simulink model "NCS_Simulation"  (R2019a)
settings: Solver=ode4  StartTime=0.0  StopTime=200  FixedStep=0.004  MaxStep=0.01  RelTol=1e-3
values from neighbouring files (symbols this model uses):
  CAN2EthernetDelay = 0.000    (= 0)    [Parameter.m]
  CycleTime_Sensor = 1/1000    (= 0.001)    [Parameter.m]
  Ethernet2CANDelay = 0.005    [Parameter.m]
  n = 0.001    [Parameter.m]
  nW_ges = 8    [Parameter.m]
  ReferenceDelay = 0.0    (= 0)    [Parameter.m]
undefined symbols (not defined in the file or in its folder): BUSCapacity, controlGate, entity, m, ReadData, ReadSize, v0
libraries: NCS_Library x250, simulink x12
(part 1 of 3)
settings Model: Creator=Moritz  LastModifiedBy=christophunterauer
settings SolverCC: InitialStep=0.01  MaxConsecutiveZCs=none  ZeroCrossControl=DisableAll  ZeroCrossAlgorithm=Adaptive
settings DataIOCC: ReturnWorkspaceOutputs=off
settings DebuggingCC: ArithmeticOperatorsInVariantConditions=warning

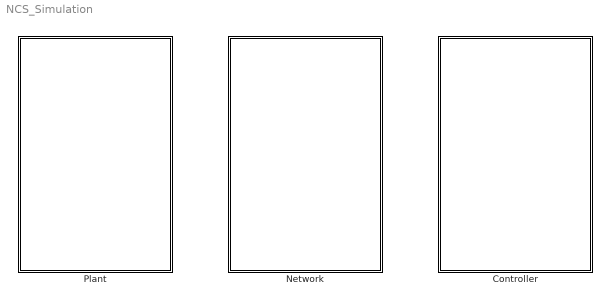
== system NCS_Simulation ==
  Controller : Subsystem
  Network : Subsystem
  Plant : Subsystem

== system NCS_Simulation/Controller ==
  note: k_P = 0.35
  Display : Display
  Display1 : Display
  Subsystem : NCS_Library/Controller/Subsystem  Scenario=Arrival  v_0=300  v_d=300
  Train Controller with PID1 : NCS_Library/Controller/Train Controller with PID  P_dyn=0.5  I_dyn=0  D_dyn=0  P_mg=1  I_mg=0  D_mg=0
  Train Controller with PID2 : NCS_Library/Controller/Train Controller with PID  P_dyn=0.5  I_dyn=0  D_dyn=0  P_mg=1  I_mg=0  D_mg=0
  tag scope: U_1=global, U_2=global
  wires:
  Subsystem/1 -> Train Controller with PID1/2, Train Controller with PID2/2  "Signal"
  Train Controller with PID1/1 -> Display1/1, [U_1]
  [Y_M_1] -> Train Controller with PID1/1  "Y_M"
  [Y_M_2] -> Train Controller with PID2/1  "Y_M"
  Train Controller with PID2/1 -> Display/1, [U_2]

== system NCS_Simulation/Network ==
  Ethernet (Line) : Subsystem  Commented=on
  Ethernet (Line) CAN : Subsystem  Commented=on
  Ethernet (Ring) CAN : Subsystem  Commented=on
  NetworkSelector : NCS_Library/Network/Applications/NetworkSelector  NetworkType=Reference  band=100 MB/s  BER=0.01  RD=0
  Reference : Subsystem

== system NCS_Simulation/Plant ==
  Network to Actuator : Subsystem
  Plant (Train) : Subsystem
  Sensor to Network : Subsystem
  wires:
  Plant (Train)/1(Sensor1) -> Sensor to Network/1(Sensor1)
  Plant (Train)/2(Sensor2) -> Sensor to Network/2(Sensor2)
  Plant (Train)/3(Sensor3) -> Sensor to Network/3(Sensor3)
  Plant (Train)/4(Sensor4) -> Sensor to Network/4(Sensor4)
  Network to Actuator/1(Actuator1) -> Plant (Train)/1(Actuator1)
  Network to Actuator/2(Actuator2) -> Plant (Train)/2(Actuator2)
  Network to Actuator/3(Actuator3) -> Plant (Train)/3(Actuator3)
  Network to Actuator/4(Actuator4) -> Plant (Train)/4(Actuator4)
  Network to Actuator/5(Actuator5) -> Plant (Train)/5(Actuator5)
  Network to Actuator/6(Actuator6) -> Plant (Train)/6(Actuator6)
  Network to Actuator/7(Actuator7) -> Plant (Train)/7(Actuator7)
  Network to Actuator/8(Actuator8) -> Plant (Train)/8(Actuator8)
  Plant (Train)/5(Sensor5) -> Sensor to Network/5(Sensor5)
  Plant (Train)/6(Sensor6) -> Sensor to Network/6(Sensor6)
  Plant (Train)/7(Sensor7) -> Sensor to Network/7(Sensor7)
  Plant (Train)/8(Sensor8) -> Sensor to Network/8(Sensor8)

== system NCS_Simulation/Network/Ethernet (Line) ==
  Consist 1 : Subsystem
  Consist 2 : Subsystem
  Mux Consist : NCS_Library/Network/Applications/Multiplexer/Mux Consist  SystemSampleTime=-1
  tag scope: Ethernet=global
  wires:
  Consist 2/1(out2) -> Mux Consist/2
  Mux Consist/1 -> [Ethernet]
  Consist 1/1(out1) -> Mux Consist/1

== system NCS_Simulation/Network/Ethernet (Line) CAN ==
  Consist 1 : Subsystem
  Consist 2 : Subsystem
  Mux Consist : NCS_Library/Network/Applications/Multiplexer/Mux Consist  SystemSampleTime=-1
  tag scope: CAN=global
  wires:
  Consist 1/1(out1) -> Mux Consist/1
  Mux Consist/1 -> [CAN]
  Consist 2/1(out2) -> Mux Consist/2

== system NCS_Simulation/Network/Ethernet (Ring) CAN ==
  Consist 1 : Subsystem
  Consist 2 : Subsystem
  Mux Consist : NCS_Library/Network/Applications/Multiplexer/Mux Consist  SystemSampleTime=-1
  tag scope: EthernetCAN_Ring=global
  wires:
  Consist 1/1(out1) -> Mux Consist/1
  Mux Consist/1 -> [EthernetCAN_Ring]
  Consist 2/1(out2) -> Mux Consist/2

== system NCS_Simulation/Network/Reference ==
  note: Consist 2
  note: Consist 1
  Mux : NCS_Library/Network/Applications/Multiplexer/Mux  SystemSampleTime=-1
  Mux Consist : NCS_Library/Network/Applications/Multiplexer/Mux Consist  SystemSampleTime=-1
  Mux Reference Y_M : NCS_Library/Network/Applications/Multiplexer/Mux Reference Y_M  SystemSampleTime=-1
  Mux Reference Y_M1 : NCS_Library/Network/Applications/Multiplexer/Mux Reference Y_M  SystemSampleTime=-1
  Mux U : NCS_Library/Network/Applications/Multiplexer/Mux U  SystemSampleTime=-1
  Mux U1 : NCS_Library/Network/Applications/Multiplexer/Mux U  SystemSampleTime=-1
  Mux2 : NCS_Library/Network/Applications/Multiplexer/Mux  SystemSampleTime=-1
  Transport Delay : TransportDelay  DelayTime=ReferenceDelay
  tag scope: Reference=global
  wires:
  Transport Delay/1 -> [Reference]
  [y_M_1] -> Mux Reference Y_M/1
  [y_M_2] -> Mux Reference Y_M/2
  [y_M_3] -> Mux Reference Y_M/3
  [y_M_4] -> Mux Reference Y_M/4
  [y_M_6] -> Mux Reference Y_M1/2
  [y_M_7] -> Mux Reference Y_M1/3
  [y_M_5] -> Mux Reference Y_M1/1
  [y_M_8] -> Mux Reference Y_M1/4
  [U_1] -> Mux U/1
  Mux Reference Y_M/1 -> Mux/1  "Y_M"
  Mux Reference Y_M1/1 -> Mux2/1
  [U_2] -> Mux U1/1
  Mux Consist/1 -> Transport Delay/1
  Mux/1 -> Mux Consist/1
  Mux2/1 -> Mux Consist/2
  Mux U/1 -> Mux/2
  Mux U1/1 -> Mux2/2

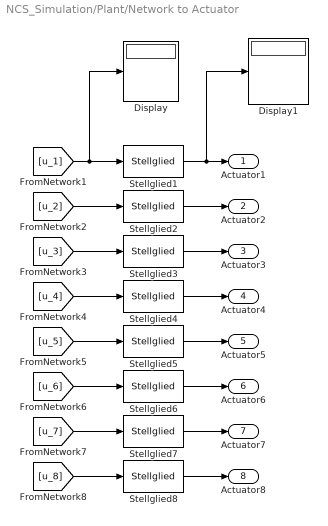
== system NCS_Simulation/Plant/Network to Actuator ==
  Display : Display
  Display1 : Display
  Stellglied{1..8} (8 alike) : NCS_Library/Plant (Train)/Stellglied  SystemSampleTime=-1
  Actuator1 : Outport
  Actuator2 : Outport  Port=2
  Actuator3 : Outport  Port=3
  Actuator4 : Outport  Port=4
  Actuator5 : Outport  Port=5
  Actuator6 : Outport  Port=6
  Actuator7 : Outport  Port=7
  Actuator8 : Outport  Port=8
  wires:
  [u_1] -> Display/1, Stellglied1/1
  [u_4] -> Stellglied4/1
  [u_2] -> Stellglied2/1
  [u_3] -> Stellglied3/1
  Stellglied4/1 -> Actuator4/1
  Stellglied1/1 -> Display1/1, Actuator1/1
  Stellglied2/1 -> Actuator2/1
  Stellglied3/1 -> Actuator3/1
  Stellglied7/1 -> Actuator7/1
  Stellglied6/1 -> Actuator6/1
  Stellglied8/1 -> Actuator8/1
  Stellglied5/1 -> Actuator5/1
  [u_7] -> Stellglied7/1
  [u_5] -> Stellglied5/1
  [u_6] -> Stellglied6/1
  [u_8] -> Stellglied8/1

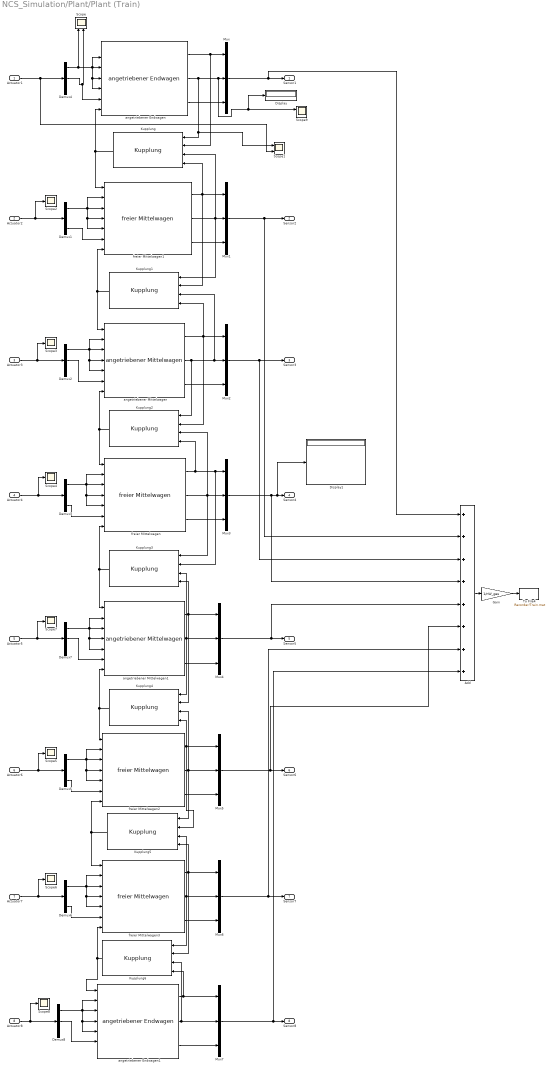
== system NCS_Simulation/Plant/Plant (Train) ==
  Actuator1 : Inport
  Actuator2 : Inport  Port=2
  Actuator3 : Inport  Port=3
  Actuator4 : Inport  Port=4
  Actuator5 : Inport  Port=5
  Actuator6 : Inport  Port=6
  Actuator7 : Inport  Port=7
  Actuator8 : Inport  Port=8
  Add : Sum  Inputs=++++++++
  Demux{1..8} (8 alike) : Demux  Outputs=3
  Display : Display
  Display1 : Display
  Gain : Gain  Gain=1/nW_ges
  Kupplung{,1..6} (7 alike) : NCS_Library/Plant (Train)/Kupplung  SystemSampleTime=-1
  Mux{,1..7} (8 alike) : Mux  Inputs=3
  Scope : Scope  NumInputPorts=2
  Scope1 : Scope  NumInputPorts=2
  Scope{2..8} (7 alike) : Scope
  Scope9 : Scope  NumInputPorts=2
  To File4 : ToFile  Filename=Recorder/Train.mat  MatrixName=Recorder
      mask Display: disp('Recorder')
  angetriebener Endwagen : NCS_Library/Plant (Train)/angetriebener Endwagen  SystemSampleTime=-1
  angetriebener Endwagen1 : NCS_Library/Plant (Train)/angetriebener Endwagen  SystemSampleTime=-1
  angetriebener Mittelwagen : NCS_Library/Plant (Train)/angetriebener Mittelwagen  SystemSampleTime=-1
  angetriebener Mittelwagen1 : NCS_Library/Plant (Train)/angetriebener Mittelwagen  SystemSampleTime=-1
  freier Mittelwagen{,1..3} (4 alike) : NCS_Library/Plant (Train)/freier Mittelwagen  SystemSampleTime=-1
  Sensor1 : Outport
  Sensor2 : Outport  Port=2
  Sensor3 : Outport  Port=3
  Sensor4 : Outport  Port=4
  Sensor5 : Outport  Port=5
  Sensor6 : Outport  Port=6
  Sensor7 : Outport  Port=7
  Sensor8 : Outport  Port=8
  wires:
  Kupplung/1 -> angetriebener Endwagen/7, freier Mittelwagen1/1
  Kupplung2/1 -> freier Mittelwagen/1, angetriebener Mittelwagen/7
  Kupplung1/1 -> freier Mittelwagen1/7, angetriebener Mittelwagen/1
  Demux1/1 -> freier Mittelwagen1/2, freier Mittelwagen1/5, freier Mittelwagen1/4, freier Mittelwagen1/3
  Demux1/3 -> freier Mittelwagen1/6
  Mux/1 -> Add/1, Sensor1/1
  angetriebener Endwagen/2 -> Scope1/1, Kupplung/1, Display/1, Scope9/1, Mux/2
  angetriebener Endwagen/1 -> Kupplung/2, Mux/1
  angetriebener Endwagen/3 -> Mux/3
  freier Mittelwagen1/1 -> Kupplung1/2, Kupplung/4, Mux1/1
  freier Mittelwagen1/2 -> Kupplung1/1, Kupplung/3, Mux1/2
  freier Mittelwagen1/3 -> Mux1/3
  angetriebener Mittelwagen/1 -> Kupplung2/2, Kupplung1/4, Mux2/1
  angetriebener Mittelwagen/2 -> Kupplung2/1, Kupplung1/3, Mux2/2
  angetriebener Mittelwagen/3 -> Mux2/3
  freier Mittelwagen/1 -> Kupplung2/4, Kupplung3/2, Mux3/1
  freier Mittelwagen/2 -> Kupplung3/1, Kupplung2/3, Mux3/2
  freier Mittelwagen/3 -> Mux3/3
  Mux1/1 -> Add/2, Sensor2/1
  Mux2/1 -> Add/3, Sensor3/1
  Mux3/1 -> Add/4, Display1/1, Sensor4/1
  Actuator2/1 -> Scope2/1, Demux1/1
  Demux2/1 -> angetriebener Mittelwagen/5, angetriebener Mittelwagen/4, angetriebener Mittelwagen/2, angetriebener Mittelwagen/3
  Actuator3/1 -> Scope3/1, Demux2/1
  Demux3/1 -> freier Mittelwagen/3, freier Mittelwagen/2, freier Mittelwagen/5, freier Mittelwagen/4
  Demux3/3 -> freier Mittelwagen/6
  Actuator4/1 -> Scope4/1, Demux3/1
  Actuator1/1 -> Scope1/2, Demux4/1
  Demux4/1 -> Scope/1, angetriebener Endwagen/2, angetriebener Endwagen/3, angetriebener Endwagen/5, angetriebener Endwagen/4
  Demux4/2 -> angetriebener Endwagen/6, Scope/2
  Add/1 -> Gain/1
  Gain/1 -> To File4/1
  angetriebener Mittelwagen1/1 -> Mux4/1, Kupplung3/4, Kupplung4/2
  angetriebener Mittelwagen1/2 -> Mux4/2, Kupplung3/3, Kupplung4/1
  Kupplung3/1 -> angetriebener Mittelwagen1/1, freier Mittelwagen/7
  Kupplung4/1 -> angetriebener Mittelwagen1/7, freier Mittelwagen2/1
  Demux5/3 -> freier Mittelwagen2/6
  Actuator6/1 -> Scope5/1, Demux5/1
  Demux5/1 -> freier Mittelwagen2/3, freier Mittelwagen2/2, freier Mittelwagen2/5, freier Mittelwagen2/4
  Demux6/3 -> freier Mittelwagen3/6
  Actuator7/1 -> Scope6/1, Demux6/1
  Demux6/1 -> freier Mittelwagen3/2, freier Mittelwagen3/3, freier Mittelwagen3/4, freier Mittelwagen3/5
  Kupplung5/1 -> freier Mittelwagen3/1, freier Mittelwagen2/7
  Kupplung6/1 -> freier Mittelwagen3/7, angetriebener Endwagen1/1
  freier Mittelwagen3/1 -> Mux6/1, Kupplung5/4, Kupplung6/2
  freier Mittelwagen3/2 -> Mux6/2, Kupplung5/3, Kupplung6/1
  freier Mittelwagen2/2 -> Mux5/2, Kupplung5/1, Kupplung4/3
  freier Mittelwagen2/1 -> Mux5/1, Kupplung5/2, Kupplung4/4
  Actuator5/1 -> Scope7/1, Demux7/1
  Demux7/1 -> angetriebener Mittelwagen1/2, angetriebener Mittelwagen1/3, angetriebener Mittelwagen1/5, angetriebener Mittelwagen1/4
  Demux8/1 -> angetriebener Endwagen1/2, angetriebener Endwagen1/3, angetriebener Endwagen1/5, angetriebener Endwagen1/4
  Actuator8/1 -> Scope8/1, Demux8/1
  angetriebener Endwagen1/1 -> Mux7/1, Kupplung6/4
  Mux4/1 -> Add/5, Sensor5/1
  angetriebener Mittelwagen1/3 -> Mux4/3
  freier Mittelwagen2/3 -> Mux5/3
  Mux5/1 -> Add/6, Sensor6/1
  freier Mittelwagen3/3 -> Mux6/3
  angetriebener Endwagen1/3 -> Mux7/3
  angetriebener Endwagen1/2 -> Mux7/2, Kupplung6/3
  Mux7/1 -> Add/8, Sensor8/1
  Mux6/1 -> Add/7, Sensor7/1
  Demux2/2 -> angetriebener Mittelwagen/6
  Demux7/2 -> angetriebener Mittelwagen1/6
  Demux8/2 -> angetriebener Endwagen1/6

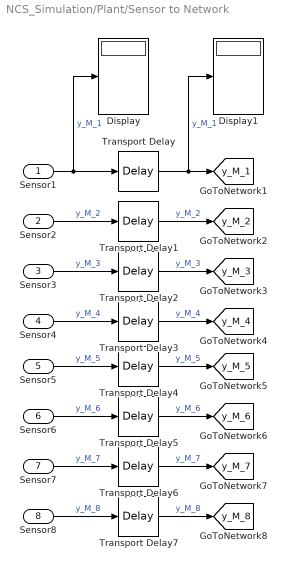
== system NCS_Simulation/Plant/Sensor to Network ==
  Sensor1 : Inport
  Sensor2 : Inport  Port=2
  Sensor3 : Inport  Port=3
  Sensor4 : Inport  Port=4
  Sensor5 : Inport  Port=5
  Sensor6 : Inport  Port=6
  Sensor7 : Inport  Port=7
  Sensor8 : Inport  Port=8
  Display : Display
  Display1 : Display
  Transport Delay{,1..7} (8 alike) : TransportDelay  DelayTime=CycleTime_Sensor  InitialOutput=[ 0 v0 0]
  tag scope: y_M_1=global, y_M_2=global, y_M_3=global, y_M_4=global, y_M_5=global, y_M_6=global, y_M_7=global, y_M_8=global
  wires:
  Sensor1/1 -> Display/1, Transport Delay/1  "y_M_1"
  Transport Delay/1 -> Display1/1, [y_M_1]  "y_M_1"
  Sensor2/1 -> Transport Delay1/1  "y_M_2"
  Sensor3/1 -> Transport Delay2/1  "y_M_3"
  Sensor4/1 -> Transport Delay3/1  "y_M_4"
  Transport Delay1/1 -> [y_M_2]  "y_M_2"
  Transport Delay2/1 -> [y_M_3]  "y_M_3"
  Transport Delay3/1 -> [y_M_4]  "y_M_4"
  Transport Delay7/1 -> [y_M_8]  "y_M_8"
  Transport Delay6/1 -> [y_M_7]  "y_M_7"
  Transport Delay5/1 -> [y_M_6]  "y_M_6"
  Sensor8/1 -> Transport Delay7/1  "y_M_8"
  Sensor7/1 -> Transport Delay6/1  "y_M_7"
  Sensor6/1 -> Transport Delay5/1  "y_M_6"
  Transport Delay4/1 -> [y_M_5]  "y_M_5"
  Sensor5/1 -> Transport Delay4/1  "y_M_5"

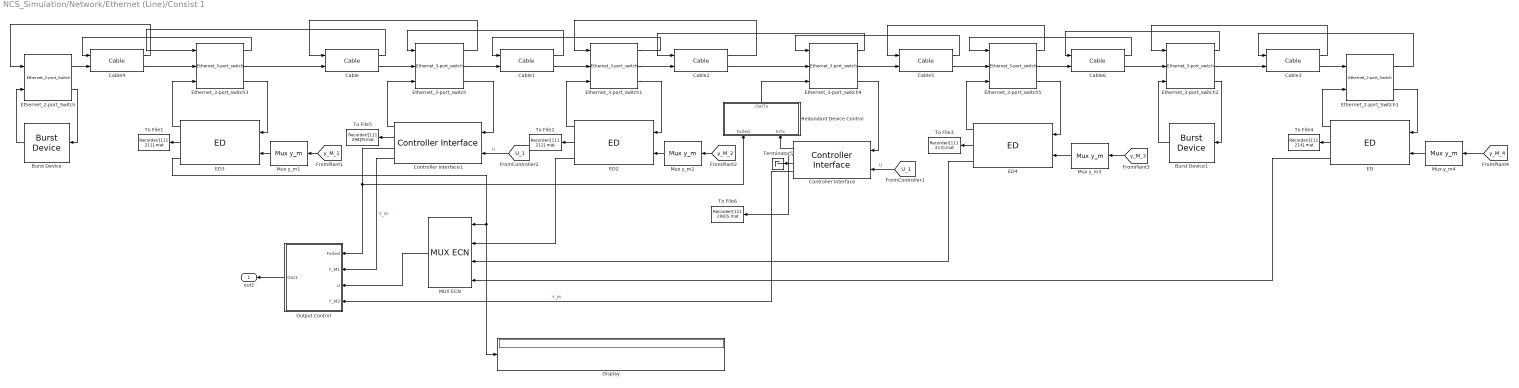
== system NCS_Simulation/Network/Ethernet (Line)/Consist 1 ==
  Burst Device : NCS_Library/Network/ETB/Burst Device  Address=[111 288]  Destination=[ 100 200]  Size=100  Port=1  ReplyAddress=[0 0]  Subscribe=[0 0; 0 0; 0 0; 0 0; 0 0]  msgType=Passive  Tx=0  Timeout=0  SDTv2=Disable  EnableToF=off  ToF=0  EnableBurst=off  ToB=0  n_Burst=0
  Burst Device1 : NCS_Library/Network/ETB/Burst Device  Address=[111 277]  Destination=[ 100 200]  Size=100  Port=1  ReplyAddress=[0 0]  Subscribe=[0 0; 0 0; 0 0; 0 0; 0 0]  msgType=Passive  Tx=0  Timeout=0  SDTv2=Disable  EnableToF=off  ToF=0  EnableBurst=off  ToB=0  n_Burst=0
  Cable{,2,4..6} (5 alike) : NCS_Library/Network/ETB/Cable  length=100  Cable=Coaxial
  Cable1 : NCS_Library/Network/ETB/Cable  length=0  Cable=Coaxial
  Cable3 : NCS_Library/Network/ETB/Cable  length=0  Cable=Coaxial
  Controller Interface : NCS_Library/Network/ETB/Controller Interface  Address=[111 298]  Sensors=[111 211; 111 212; 111 213; 111 214]  Actuators=[111 211; 111 212; 111 213; 111 214]  Size=11  EnableToF=off  ToF=0  Enable_1=on  msgType_1=Push by Controller  SDTv2_1=Disable  Tx_1=40  Enable_2=on  msgType_2=Push by Controller  SDTv2_2=Disable  Tx_2=40  Enable_3=on  msgType_3=Push by Controller  SDTv2_3=Disable  Tx_3=40  Enable_4=on  msgType_4=Push by Controller  SDTv2_4=Disable  Tx_4=40
  Controller Interface1 : NCS_Library/Network/ETB/Controller Interface  Address=[111 298]  Sensors=[111 211; 111 212; 111 213; 111 214]  Actuators=[111 211; 111 212; 111 213; 111 214]  Size=11  EnableToF=off  ToF=0  Enable_1=on  msgType_1=Push by Controller  SDTv2_1=Disable  Tx_1=40  Enable_2=on  msgType_2=Push by Controller  SDTv2_2=Disable  Tx_2=40  Enable_3=on  msgType_3=Push by Controller  SDTv2_3=Disable  Tx_3=40  Enable_4=on  msgType_4=Push by Controller  SDTv2_4=Disable  Tx_4=40
  Display : Display
  ED : NCS_Library/Network/ETB/ED  Address=[111 214]  Destination=[ 111 200 ]  Port=4  ReplyAddress=[0 0]  Size=11  Subscribe=[111 299; 111 298; 0 0; 0 0; 0 0]  msgType=Push cyclical  Tx=40  Timeout=2  SDTv2=Disable  EnableToF=off  ToF=0
  ED2 : NCS_Library/Network/ETB/ED  Address=[111 212]  Destination=[ 111 200]  Port=2  ReplyAddress=[0 0]  Size=11  Subscribe=[111 299; 111 298; 0 0; 0 0; 0 0]  msgType=Push cyclical  Tx=40  Timeout=2  SDTv2=Disable  EnableToF=off  ToF=0
  ED3 : NCS_Library/Network/ETB/ED  Address=[111 211]  Destination=[ 111 200]  Port=1  ReplyAddress=[0 0]  Size=11  Subscribe=[111 299; 111 298; 0 0; 0 0; 0 0]  msgType=Push cyclical  Tx=40  Timeout=2  SDTv2=Disable  EnableToF=off  ToF=5
  ED4 : NCS_Library/Network/ETB/ED  Address=[111 213]  Destination=[ 111 200]  Port=3  ReplyAddress=[0 0]  Size=11  Subscribe=[111 299; 111 298; 0 0; 0 0; 0 0]  msgType=Push cyclical  Tx=40  Timeout=2  SDTv2=Disable  EnableToF=off  ToF=0
  Ethernet_2-port_Switch : NCS_Library/Network/ETB/Ethernet_2-port_Switch  addstore=10  bandc=10^8  buffer_size=120000  cable_node=10  cable_LR=10
  Ethernet_2-port_Switch1 : NCS_Library/Network/ETB/Ethernet_2-port_Switch  addstore=10  bandc=10^8  buffer_size=120000  cable_node=10  cable_LR=10
  Ethernet_3-port_switch{,1..5} (6 alike) : NCS_Library/Network/ETB/Ethernet_3-port_switch  addstore=5  bandc=10^8  buffer_size=180000  cable_node=10  cable_L=10  cable_R=10
  MUX ECN : NCS_Library/Network/Applications/Multiplexer/MUX ECN  SystemSampleTime=-1
  Mux y_m{1..4} (4 alike) : NCS_Library/Network/Applications/Multiplexer/Mux y_m  SystemSampleTime=-1
  Output Control : Subsystem
  Redundant Device Control : Subsystem
  Terminator5 : Terminator
  To File1 : ToFile  Filename=Recorder/[111 211].mat  MatrixName=ED  SaveFormat=Timeseries
  To File2 : ToFile  Filename=Recorder/[111 212].mat  MatrixName=ED  SaveFormat=Timeseries
  To File3 : ToFile  Filename=Recorder/[111 213].mat  MatrixName=ED  SaveFormat=Timeseries
  To File4 : ToFile  Filename=Recorder/[111 214].mat  MatrixName=ED  SaveFormat=Timeseries
  To File5 : ToFile  Filename=Recorder/[111 298]M.mat  MatrixName=ED  SaveFormat=Timeseries
  To File6 : ToFile  Filename=Recorder/[111 298]S.mat  MatrixName=ED  SaveFormat=Timeseries
  out1 : Outport
  wires:
  Controller Interface1/4 -> Output Control/2(Y_M1)  "Y_M"
  Cable3/2 -> Ethernet_2-port_Switch1/1
  Cable2/1 -> Ethernet_3-port_switch1/1
  Controller Interface/1 -> Redundant Device Control/2(InTx)
  Ethernet_2-port_Switch/2 -> Burst Device/1
  Ethernet_2-port_Switch1/1 -> Cable3/1
  Burst Device/1 -> Ethernet_2-port_Switch/2
  Ethernet_3-port_switch/3 -> Controller Interface1/1
  Controller Interface1/3 -> Redundant Device Control/1(Failed), Output Control/1(Failed)
  Cable1/1 -> Ethernet_3-port_switch/1
  Controller Interface/4 -> Output Control/4(Y_M2)  "Y_M"
  Ethernet_3-port_switch/1 -> Cable/1
  Cable3/1 -> Ethernet_3-port_switch2/1
  Output Control/1(Out1) -> out1/1
  [U_1] -> Controller Interface/2  "U"
  Ethernet_3-port_switch2/2 -> Cable3/2
  Ethernet_3-port_switch1/2 -> Cable2/2
  Ethernet_3-port_switch/2 -> Cable1/2
  Cable/2 -> Ethernet_3-port_switch/2
  Cable1/2 -> Ethernet_3-port_switch1/2
  Ethernet_3-port_switch1/1 -> Cable1/1
  Controller Interface1/1 -> Ethernet_3-port_switch/3
  [U_1] -> Controller Interface1/2  "U"
  ED2/1 -> Ethernet_3-port_switch1/3
  Ethernet_3-port_switch1/3 -> ED2/1
  ED2/2 -> To File2/1
  [y_M_2] -> Mux y_m2/1
  Ethernet_3-port_switch3/2 -> Cable/2
  Cable/1 -> Ethernet_3-port_switch3/1
  ED3/1 -> Ethernet_3-port_switch3/3
  Ethernet_3-port_switch3/3 -> ED3/1
  Ethernet_2-port_Switch/1 -> Cable4/2
  Cable4/2 -> Ethernet_3-port_switch3/2
  Cable4/1 -> Ethernet_2-port_Switch/1
  Ethernet_3-port_switch3/1 -> Cable4/1
  Cable2/2 -> Ethernet_3-port_switch4/2
  Ethernet_3-port_switch4/2 -> Cable5/2
  Cable5/2 -> Ethernet_3-port_switch5/2
  Redundant Device Control/1(OutTx) -> Ethernet_3-port_switch4/3
  Ethernet_3-port_switch4/3 -> Controller Interface/1
  ED4/1 -> Ethernet_3-port_switch5/3
  Ethernet_3-port_switch5/3 -> ED4/1
  [y_M_3] -> Mux y_m3/1
  ED4/2 -> To File3/1
  Ethernet_3-port_switch5/2 -> Cable6/2
  Cable6/2 -> Ethernet_3-port_switch2/2
  Ethernet_3-port_switch4/1 -> Cable2/1
  Cable5/1 -> Ethernet_3-port_switch4/1
  Ethernet_3-port_switch5/1 -> Cable5/1
  Ethernet_3-port_switch2/3 -> Burst Device1/1
  Burst Device1/1 -> Ethernet_3-port_switch2/3
  Cable6/1 -> Ethernet_3-port_switch5/1
  Ethernet_3-port_switch2/1 -> Cable6/1
  ED/1 -> Ethernet_2-port_Switch1/2
  Ethernet_2-port_Switch1/2 -> ED/1
  ED/2 -> To File4/1
  [y_M_4] -> Mux y_m4/1
  [y_M_1] -> Mux y_m1/1
  ED3/2 -> To File1/1
  Controller Interface/2 -> To File6/1
  MUX ECN/1 -> Output Control/3(U)
  ED3/3 -> Display/1, MUX ECN/1
  ED2/3 -> MUX ECN/2
  ED4/3 -> MUX ECN/3
  ED/3 -> MUX ECN/4
  Mux y_m1/1 -> ED3/2
  Mux y_m4/1 -> ED/2
  Mux y_m3/1 -> ED4/2
  Mux y_m2/1 -> ED2/2
  Controller Interface/3 -> Terminator5/1
  Controller Interface1/2 -> To File5/1

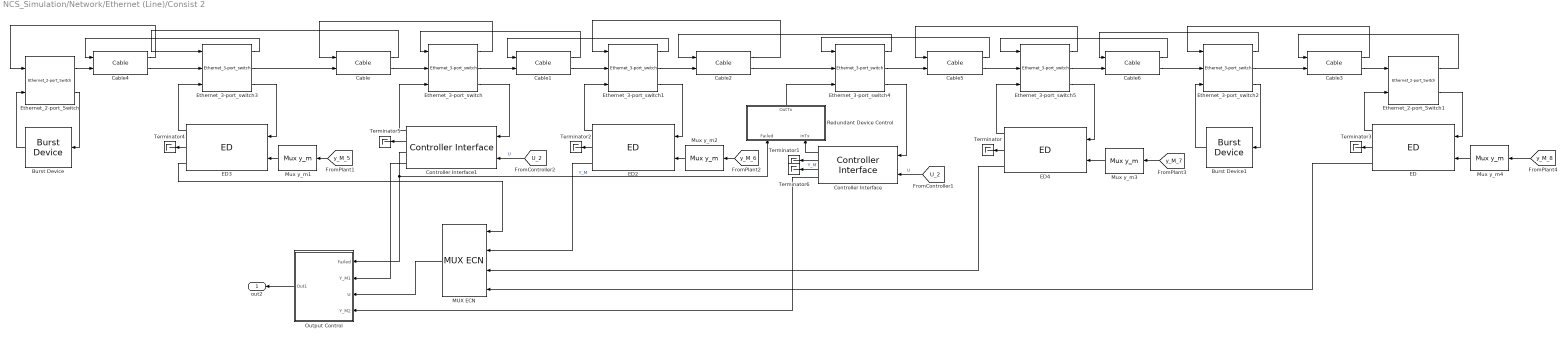
== system NCS_Simulation/Network/Ethernet (Line)/Consist 2 ==
  Burst Device : NCS_Library/Network/ETB/Burst Device  Address=[111 288]  Destination=[ 100 200]  Size=100  Port=1  ReplyAddress=[0 0]  Subscribe=[0 0; 0 0; 0 0; 0 0; 0 0]  msgType=Passive  Tx=0  Timeout=0  SDTv2=Disable  EnableToF=off  ToF=0  EnableBurst=off  ToB=0  n_Burst=0
  Burst Device1 : NCS_Library/Network/ETB/Burst Device  Address=[111 277]  Destination=[ 100 200]  Size=100  Port=1  ReplyAddress=[0 0]  Subscribe=[0 0; 0 0; 0 0; 0 0; 0 0]  msgType=Passive  Tx=0  Timeout=0  SDTv2=Disable  EnableToF=off  ToF=0  EnableBurst=on  ToB=30  n_Burst=10000
  Cable{,2,4..6} (5 alike) : NCS_Library/Network/ETB/Cable  length=100  Cable=Coaxial
  Cable1 : NCS_Library/Network/ETB/Cable  length=0  Cable=Coaxial
  Cable3 : NCS_Library/Network/ETB/Cable  length=0  Cable=Coaxial
  Controller Interface : NCS_Library/Network/ETB/Controller Interface  Address=[111 298]  Sensors=[111 211; 111 212; 111 213; 111 214]  Actuators=[111 211; 111 212; 111 213; 111 214]  Size=11  EnableToF=off  ToF=0  Enable_1=on  msgType_1=Push by Controller  SDTv2_1=Disable  Tx_1=0.1  Enable_2=on  msgType_2=Push by Controller  SDTv2_2=Disable  Tx_2=0.1  Enable_3=on  msgType_3=Push by Controller  SDTv2_3=Disable  Tx_3=0.1  Enable_4=on  msgType_4=Push by Controller  SDTv2_4=Disable  Tx_4=0.1
  Controller Interface1 : NCS_Library/Network/ETB/Controller Interface  Address=[111 299]  Sensors=[111 211; 111 212; 111 213; 111 214]  Actuators=[111 211; 111 212; 111 213; 111 214]  Size=11  EnableToF=off  ToF=0  Enable_1=on  msgType_1=Push by Controller  SDTv2_1=Disable  Tx_1=40  Enable_2=on  msgType_2=Push by Controller  SDTv2_2=Disable  Tx_2=40  Enable_3=on  msgType_3=Push by Controller  SDTv2_3=Disable  Tx_3=40  Enable_4=on  msgType_4=Push by Controller  SDTv2_4=Disable  Tx_4=40
  ED : NCS_Library/Network/ETB/ED  Address=[111 214]  Destination=[ 111 200 ]  Port=4  ReplyAddress=[0 0]  Size=11  Subscribe=[111 299; 111 298; 0 0; 0 0; 0 0]  msgType=Push cyclical  Tx=40  Timeout=2  SDTv2=Disable  EnableToF=off  ToF=0
  ED2 : NCS_Library/Network/ETB/ED  Address=[111 212]  Destination=[ 111 200]  Port=2  ReplyAddress=[0 0]  Size=11  Subscribe=[111 299; 111 298; 0 0; 0 0; 0 0]  msgType=Push cyclical  Tx=40  Timeout=2  SDTv2=Disable  EnableToF=off  ToF=0
  ED3 : NCS_Library/Network/ETB/ED  Address=[111 211]  Destination=[ 111 200]  Port=1  ReplyAddress=[0 0]  Size=11  Subscribe=[111 299; 111 298; 0 0; 0 0; 0 0]  msgType=Push cyclical  Tx=40  Timeout=2  SDTv2=Disable  EnableToF=off  ToF=0
  ED4 : NCS_Library/Network/ETB/ED  Address=[111 213]  Destination=[ 111 200]  Port=3  ReplyAddress=[0 0]  Size=11  Subscribe=[111 299; 111 298; 0 0; 0 0; 0 0]  msgType=Push cyclical  Tx=40  Timeout=2  SDTv2=Disable  EnableToF=off  ToF=0
  Ethernet_2-port_Switch : NCS_Library/Network/ETB/Ethernet_2-port_Switch  addstore=10  bandc=10^8  buffer_size=120000  cable_node=10  cable_LR=10
  Ethernet_2-port_Switch1 : NCS_Library/Network/ETB/Ethernet_2-port_Switch  addstore=10  bandc=10^8  buffer_size=120000  cable_node=10  cable_LR=10
  Ethernet_3-port_switch{,1..5} (6 alike) : NCS_Library/Network/ETB/Ethernet_3-port_switch  addstore=5  bandc=10^8  buffer_size=180000  cable_node=10  cable_L=10  cable_R=10
  MUX ECN : NCS_Library/Network/Applications/Multiplexer/MUX ECN  SystemSampleTime=-1
  Mux y_m{1..4} (4 alike) : NCS_Library/Network/Applications/Multiplexer/Mux y_m  SystemSampleTime=-1
  Output Control : Subsystem
  Redundant Device Control : Subsystem
  Terminator{,1..6} (7 alike) : Terminator
  out2 : Outport
  wires:
  Cable3/2 -> Ethernet_2-port_Switch1/1
  Cable2/1 -> Ethernet_3-port_switch1/1
  Controller Interface/1 -> Redundant Device Control/2(InTx)
  Ethernet_2-port_Switch/2 -> Burst Device/1
  Ethernet_2-port_Switch1/1 -> Cable3/1
  Burst Device/1 -> Ethernet_2-port_Switch/2
  Ethernet_3-port_switch/3 -> Controller Interface1/1
  Cable1/1 -> Ethernet_3-port_switch/1
  Ethernet_3-port_switch/1 -> Cable/1
  Cable3/1 -> Ethernet_3-port_switch2/1
  Output Control/1(Out1) -> out2/1
  [U_2] -> Controller Interface/2  "U"
  Ethernet_3-port_switch2/2 -> Cable3/2
  Ethernet_3-port_switch1/2 -> Cable2/2
  Ethernet_3-port_switch/2 -> Cable1/2
  Cable/2 -> Ethernet_3-port_switch/2
  Cable1/2 -> Ethernet_3-port_switch1/2
  Ethernet_3-port_switch1/1 -> Cable1/1
  Controller Interface1/1 -> Ethernet_3-port_switch/3
  [U_2] -> Controller Interface1/2  "U"
  ED2/1 -> Ethernet_3-port_switch1/3
  Ethernet_3-port_switch1/3 -> ED2/1
  ED2/2 -> Terminator2/1
  [y_M_6] -> Mux y_m2/1
  Ethernet_3-port_switch3/2 -> Cable/2
  Cable/1 -> Ethernet_3-port_switch3/1
  ED3/1 -> Ethernet_3-port_switch3/3
  Ethernet_3-port_switch3/3 -> ED3/1
  Ethernet_2-port_Switch/1 -> Cable4/2
  Cable4/2 -> Ethernet_3-port_switch3/2
  Cable4/1 -> Ethernet_2-port_Switch/1
  Ethernet_3-port_switch3/1 -> Cable4/1
  Cable2/2 -> Ethernet_3-port_switch4/2
  Ethernet_3-port_switch4/2 -> Cable5/2
  Cable5/2 -> Ethernet_3-port_switch5/2
  Redundant Device Control/1(OutTx) -> Ethernet_3-port_switch4/3
  Ethernet_3-port_switch4/3 -> Controller Interface/1
  ED4/1 -> Ethernet_3-port_switch5/3
  Ethernet_3-port_switch5/3 -> ED4/1
  [y_M_7] -> Mux y_m3/1
  ED4/2 -> Terminator/1
  Ethernet_3-port_switch5/2 -> Cable6/2
  Cable6/2 -> Ethernet_3-port_switch2/2
  Ethernet_3-port_switch4/1 -> Cable2/1
  Cable5/1 -> Ethernet_3-port_switch4/1
  Ethernet_3-port_switch5/1 -> Cable5/1
  Ethernet_3-port_switch2/3 -> Burst Device1/1
  Burst Device1/1 -> Ethernet_3-port_switch2/3
  Cable6/1 -> Ethernet_3-port_switch5/1
  Ethernet_3-port_switch2/1 -> Cable6/1
  ED/1 -> Ethernet_2-port_Switch1/2
  Ethernet_2-port_Switch1/2 -> ED/1
  ED/2 -> Terminator3/1
  [y_M_8] -> Mux y_m4/1
  [y_M_5] -> Mux y_m1/1
  ED3/2 -> Terminator4/1
  Controller Interface/2 -> Terminator1/1
  MUX ECN/1 -> Output Control/3(U)
  ED3/3 -> MUX ECN/1
  ED2/3 -> MUX ECN/2
  ED4/3 -> MUX ECN/3
  ED/3 -> MUX ECN/4
  Mux y_m1/1 -> ED3/2
  Mux y_m4/1 -> ED/2
  Mux y_m3/1 -> ED4/2
  Mux y_m2/1 -> ED2/2
  Controller Interface1/4 -> Output Control/2(Y_M1)
  Controller Interface1/3 -> Output Control/1(Failed), Redundant Device Control/1(Failed)  "Y_M"
  Controller Interface1/2 -> Terminator5/1
  Controller Interface/4 -> Output Control/4(Y_M2)
  Controller Interface/3 -> Terminator6/1  "Y_M"

== system NCS_Simulation/Network/Ethernet (Line) CAN/Consist 1 ==
  Burst Device : NCS_Library/Network/ETB/Burst Device  Address=[111 299]  Destination=[ 100 200]  Port=1  ReplyAddress=[0 0]  Subscribe=[0 0; 0 0; 0 0; 0 0; 0 0]  msgType=Passive  Tx=0  Timeout=0  SDTv2=Disable  EnableToF=off  ToF=0  EnableBurst=off  ToB=0  n_Burst=0
  Burst Device1 : NCS_Library/Network/ETB/Burst Device  Address=[111 298]  Destination=[ 100 200]  Port=1  ReplyAddress=[0 0]  Subscribe=[0 0; 0 0; 0 0; 0 0; 0 0]  msgType=Passive  Tx=0  Timeout=0  SDTv2=Disable  EnableToF=off  ToF=0  EnableBurst=off  ToB=0  n_Burst=0
  Bus Selector : BusSelector  OutputSignals=#Receive
  Cable{,1..3} (4 alike) : NCS_Library/Network/ETB/Cable  length=0  Cable=Coaxial
  ED : NCS_Library/Network/ETB/ED  Address=[111 212]  Destination=[111 211]  Port=1  ReplyAddress=[0 0]  Size=11  Subscribe=[111 211; 0 0; 0 0; 0 0; 0 0]  msgType=Passive  Tx=0.1  Timeout=inf  SDTv2=Disable  EnableToF=on  ToF=6
  ED1 : NCS_Library/Network/ETB/ED  Address=[111 213]  Destination=[111 211]  Port=1  ReplyAddress=[0 0]  Size=11  Subscribe=[111 211; 0 0; 0 0; 0 0; 0 0]  msgType=Passive  Tx=0.1  Timeout=inf  SDTv2=Disable  EnableToF=off  ToF=0.5
  Ethernet_2-port_Switch : NCS_Library/Network/ETB/Ethernet_2-port_Switch  addstore=10  bandc=10^8  buffer_size=120000  cable_node=10  cable_LR=10
  Ethernet_2-port_Switch1 : NCS_Library/Network/ETB/Ethernet_2-port_Switch  addstore=10  bandc=10^8  buffer_size=120000  cable_node=10  cable_LR=10
  Ethernet_3-port_switch : NCS_Library/Network/ETB/Ethernet_3-port_switch  addstore=5  bandc=10^8  buffer_size=180000  cable_node=10  cable_L=10  cable_R=10
  Ethernet_3-port_switch1 : NCS_Library/Network/ETB/Ethernet_3-port_switch  addstore=5  bandc=10^8  buffer_size=180000  cable_node=10  cable_L=10  cable_R=10
  Ethernet_3-port_switch2 : NCS_Library/Network/ETB/Ethernet_3-port_switch  addstore=5  bandc=10^8  buffer_size=180000  cable_node=10  cable_L=10  cable_R=10
  Fieldbus 1 : Subsystem
  Output Control : Subsystem
  Redundant Device Control : Subsystem
  Terminator1 : Terminator
  out1 : Outport
  wires:
  [U_1] -> ED/2  "U"
  ED/1 -> Ethernet_3-port_switch/3
  ED/2 -> Bus Selector/1
  ED1/2 -> Terminator1/1
  Ethernet_3-port_switch1/1 -> Cable1/1
  Cable1/2 -> Ethernet_3-port_switch1/2
  Ethernet_2-port_Switch/1 -> Cable/2
  Cable/2 -> Ethernet_3-port_switch/2
  Ethernet_3-port_switch/2 -> Cable1/2
  Ethernet_3-port_switch1/2 -> Cable2/2
  Ethernet_3-port_switch2/2 -> Cable3/2
  [U_1] -> ED1/2  "U"
  Output Control/1(Out1) -> out1/1
  Cable3/1 -> Ethernet_3-port_switch2/1
  Ethernet_3-port_switch/1 -> Cable/1
  Redundant Device Control/1(OutTx) -> Ethernet_3-port_switch2/3
  ED1/3 -> Output Control/4(Y_M2)  "Y_M"
  Ethernet_3-port_switch2/1 -> Cable2/1
  Ethernet_2-port_Switch1/2 -> Burst Device1/1
  Ethernet_3-port_switch1/3 -> Fieldbus 1/1(InFromEthernet)
  Fieldbus 1/1(OutToEthernet) -> Ethernet_3-port_switch1/3
  Ethernet_3-port_switch2/3 -> ED1/1
  Burst Device1/1 -> Ethernet_2-port_Switch1/2
  Cable1/1 -> Ethernet_3-port_switch/1
  Bus Selector/1 -> Output Control/1(<#Receive>), Redundant Device Control/1(<#Receive>)  "<#Receive>"
  Cable/1 -> Ethernet_2-port_Switch/1
  Ethernet_3-port_switch/3 -> ED/1
  Burst Device/1 -> Ethernet_2-port_Switch/2
  Ethernet_2-port_Switch1/1 -> Cable3/1
  Cable2/2 -> Ethernet_3-port_switch2/2
  Ethernet_2-port_Switch/2 -> Burst Device/1
  ED1/1 -> Redundant Device Control/2(InTx)
  Cable2/1 -> Ethernet_3-port_switch1/1
  Cable3/2 -> Ethernet_2-port_Switch1/1
  ED/3 -> Output Control/2(Y_M1)  "Y_M"
  Fieldbus 1/2(U) -> Output Control/3(U)  "U"

== system NCS_Simulation/Network/Ethernet (Line) CAN/Consist 2 ==
  Burst Device : NCS_Library/Network/ETB/Burst Device  Address=[111 299]  Destination=[ 100 200]  Port=1  ReplyAddress=[0 0]  Subscribe=[0 0; 0 0; 0 0; 0 0; 0 0]  msgType=Passive  Tx=0  Timeout=0  SDTv2=Disable  EnableToF=off  ToF=0  EnableBurst=off  ToB=0  n_Burst=0
  Burst Device1 : NCS_Library/Network/ETB/Burst Device  Address=[111 298]  Destination=[ 100 200]  Port=1  ReplyAddress=[0 0]  Subscribe=[0 0; 0 0; 0 0; 0 0; 0 0]  msgType=Passive  Tx=0  Timeout=0  SDTv2=Disable  EnableToF=off  ToF=0  EnableBurst=off  ToB=0  n_Burst=0
  Bus Selector : BusSelector  OutputSignals=#Receive
  Cable{,1..3} (4 alike) : NCS_Library/Network/ETB/Cable  length=0  Cable=Coaxial
  ED : NCS_Library/Network/ETB/ED  Address=[112 212]  Destination=[112 211]  Port=1  ReplyAddress=[0 0]  Subscribe=[112 211; 0 0; 0 0; 0 0; 0 0]  msgType=Push Continuous  Tx=0.1  Timeout=inf  SDTv2=Disable  EnableToF=off  ToF=6  EnableBurst=off  ToB=0
  ED1 : NCS_Library/Network/ETB/ED  Address=[112 213]  Destination=[112 211]  Port=1  ReplyAddress=[0 0]  Subscribe=[112 211; 0 0; 0 0; 0 0; 0 0]  msgType=Push Continuous  Tx=0.1  Timeout=inf  SDTv2=Disable  EnableToF=off  ToF=0.5  EnableBurst=off  ToB=0
  Ethernet_2-port_Switch : NCS_Library/Network/ETB/Ethernet_2-port_Switch  addstore=10  bandc=10^8  buffer_size=120000  cable_node=10  cable_LR=10
  Ethernet_2-port_Switch1 : NCS_Library/Network/ETB/Ethernet_2-port_Switch  addstore=10  bandc=10^8  buffer_size=120000  cable_node=10  cable_LR=10
  Ethernet_3-port_switch : NCS_Library/Network/ETB/Ethernet_3-port_switch  addstore=5  bandc=10^8  buffer_size=180000  cable_node=10  cable_L=10  cable_R=10
  Ethernet_3-port_switch1 : NCS_Library/Network/ETB/Ethernet_3-port_switch  addstore=5  bandc=10^8  buffer_size=180000  cable_node=10  cable_L=10  cable_R=10
  Ethernet_3-port_switch2 : NCS_Library/Network/ETB/Ethernet_3-port_switch  addstore=5  bandc=10^8  buffer_size=180000  cable_node=10  cable_L=10  cable_R=10
  Fieldbus 2 : Subsystem
  Output Control : Subsystem
  Redundant Device Control : Subsystem
  Terminator1 : Terminator
  out2 : Outport
  wires:
  Fieldbus 2/2(U) -> Output Control/3(U)  "U"
  ED/3 -> Output Control/2(Y_M1)  "Y_M"
  Cable3/2 -> Ethernet_2-port_Switch1/1
  Cable2/1 -> Ethernet_3-port_switch1/1
  ED1/1 -> Redundant Device Control/2(InTx)
  Ethernet_2-port_Switch/2 -> Burst Device/1
  Cable2/2 -> Ethernet_3-port_switch2/2
  Ethernet_2-port_Switch1/1 -> Cable3/1
  Burst Device/1 -> Ethernet_2-port_Switch/2
  Ethernet_3-port_switch/3 -> ED/1
  Cable/1 -> Ethernet_2-port_Switch/1
  Bus Selector/1 -> Redundant Device Control/1(<#Receive>), Output Control/1(<#Receive>)  "<#Receive>"
  Cable1/1 -> Ethernet_3-port_switch/1
  Burst Device1/1 -> Ethernet_2-port_Switch1/2
  Ethernet_3-port_switch2/3 -> ED1/1
  Fieldbus 2/1(OutToEthernet) -> Ethernet_3-port_switch1/3
  Ethernet_3-port_switch1/3 -> Fieldbus 2/1(InFromEthernet)
  Ethernet_2-port_Switch1/2 -> Burst Device1/1
  Ethernet_3-port_switch2/1 -> Cable2/1
  ED1/3 -> Output Control/4(Y_M2)  "Y_M"
  Redundant Device Control/1(OutTx) -> Ethernet_3-port_switch2/3
  Ethernet_3-port_switch/1 -> Cable/1
  Cable3/1 -> Ethernet_3-port_switch2/1
  Output Control/1(Out1) -> out2/1
  Ethernet_3-port_switch2/2 -> Cable3/2
  Ethernet_3-port_switch1/2 -> Cable2/2
  Ethernet_3-port_switch/2 -> Cable1/2
  Cable/2 -> Ethernet_3-port_switch/2
  Ethernet_2-port_Switch/1 -> Cable/2
  Cable1/2 -> Ethernet_3-port_switch1/2
  Ethernet_3-port_switch1/1 -> Cable1/1
  ED1/2 -> Terminator1/1
  ED/2 -> Bus Selector/1
  ED/1 -> Ethernet_3-port_switch/3
  [U_2] -> ED/2  "U"
  [U_2] -> ED1/2  "U"

== system NCS_Simulation/Network/Ethernet (Ring) CAN/Consist 1 ==
  Burst Device : NCS_Library/Network/ETB/Burst Device  Address=[111 299]  Destination=[ 100 200]  Size=100  Port=1  ReplyAddress=[0 0]  Subscribe=[0 0; 0 0; 0 0; 0 0; 0 0]  msgType=Passive  T_x=0  Timeout=0  SDTv2=Disable  EnableToF=off  ToF=0  EnableBurst=off  ToB=0  Tx=0  number=1
  Burst Device1 : NCS_Library/Network/ETB/Burst Device  Address=[111 298]  Destination=[ 100 200]  Size=100  Port=1  ReplyAddress=[0 0]  Subscribe=[0 0; 0 0; 0 0; 0 0; 0 0]  msgType=Passive  T_x=0  Timeout=0  SDTv2=Disable  EnableToF=off  ToF=0  EnableBurst=off  ToB=0  Tx=0  number=1
  Cable{,1..4} (5 alike) : NCS_Library/Network/ETB/Cable  length=0  Cable=Coaxial
  Controller Interface : NCS_Library/Network/ETB/Controller Interface  Address=[144 211]  Sensors=[133 211; 0 0; 0 0; 0 0]  Actuators=[133 211; 0 0; 0 0; 0 0]  Size=11  EnableToF=off  ToF=0  Enable_1=on  msgType_1=Push by Controller  SDTv2_1=Disable  Tx_1=0.1  Enable_2=off  msgType_2=Push by Controller  SDTv2_2=Disable  Tx_2=0  Enable_3=off  msgType_3=Push by Controller  SDTv2_3=Disable  Tx_3=0  Enable_4=off  msgType_4=Push by Controller  SDTv2_4=Disable  Tx_4=0
  Controller Interface1 : NCS_Library/Network/ETB/Controller Interface  Address=[122 211]  Sensors=[133 211; 0 0; 0 0; 0 0]  Actuators=[133 211; 0 0; 0 0; 0 0]  Size=11  EnableToF=off  ToF=0  Enable_1=on  msgType_1=Push by Controller  SDTv2_1=Disable  Tx_1=0.1  Enable_2=off  msgType_2=Push by Controller  SDTv2_2=Disable  Tx_2=0.1  Enable_3=off  msgType_3=Push by Controller  SDTv2_3=Disable  Tx_3=0  Enable_4=off  msgType_4=Push by Controller  SDTv2_4=Disable  Tx_4=0
  Fieldbus 1 : Subsystem
  Output Control : Subsystem
  Redundant Device Control1 : Subsystem
  Subsystem1 : NCS_Library/Network/ETB/Subsystem2  RouterID=2  SubnetIDa=112  SubnetIDb=123  SubnetIDc=122  CycleTime_Router=0.05  EnableToF=off  ToF=0
  Subsystem2 : NCS_Library/Network/ETB/Subsystem2  RouterID=1  SubnetIDa=151  SubnetIDb=112  SubnetIDc=111  CycleTime_Router=0.05  EnableToF=off  ToF=0
  Subsystem3 : NCS_Library/Network/ETB/Subsystem2  RouterID=3  SubnetIDa=123  SubnetIDb=134  SubnetIDc=133  CycleTime_Router=0.05  EnableToF=off  ToF=0
  Subsystem4 : NCS_Library/Network/ETB/Subsystem2  RouterID=4  SubnetIDa=134  SubnetIDb=145  SubnetIDc=144  CycleTime_Router=0.05  EnableToF=off  ToF=0
  Subsystem5 : NCS_Library/Network/ETB/Subsystem2  RouterID=5  SubnetIDa=145  SubnetIDb=151  SubnetIDc=155  CycleTime_Router=0.05  EnableToF=off  ToF=0
  Terminator1 : Terminator
  Terminator2 : Terminator
  Terminator3 : Terminator
  out1 : Outport
  wires:
  [U_1] -> Controller Interface1/2  "U"
  Controller Interface/2 -> Terminator1/1
  [U_1] -> Controller Interface/2  "U"
  Output Control/1(Out1) -> out1/1
  Controller Interface/4 -> Output Control/4(Y_M2)  "Y_M"
  Subsystem5/3 -> Burst Device1/1
  Burst Device1/1 -> Subsystem5/3
  Controller Interface1/3 -> Redundant Device Control1/1(Failed), Output Control/1(Failed)
  Controller Interface/1 -> Redundant Device Control1/2(InTx)
  Controller Interface1/4 -> Output Control/2(Y_M1)  "Y_M"
  Fieldbus 1/2(U) -> Output Control/3(U)  "U"
  Subsystem2/3 -> Burst Device/1
  Burst Device/1 -> Subsystem2/3
  Cable/2 -> Subsystem1/1
  Controller Interface1/1 -> Subsystem1/3
  Subsystem1/3 -> Controller Interface1/1
  Fieldbus 1/1(OutToEthernet) -> Subsystem3/3
  Subsystem3/3 -> Fieldbus 1/1(InFromEthernet)
  Redundant Device Control1/1(OutTx) -> Subsystem4/3
  Subsystem4/3 -> Controller Interface/1
  Subsystem4/2 -> Cable3/2
  Cable3/2 -> Subsystem5/1
  Subsystem5/1 -> Cable3/1
  Cable3/1 -> Subsystem4/2
  Subsystem3/2 -> Cable2/2
  Cable2/2 -> Subsystem4/1
  Subsystem4/1 -> Cable2/1
  Subsystem3/1 -> Cable1/1
  Subsystem1/2 -> Cable1/2
  Cable1/1 -> Subsystem1/2
  Subsystem2/2 -> Cable/2
  Subsystem1/1 -> Cable/1
  Cable/1 -> Subsystem2/2
  Subsystem5/2 -> Cable4/2
  Cable4/1 -> Subsystem5/2
  Subsystem2/1 -> Cable4/1
  Cable4/2 -> Subsystem2/1
  Controller Interface/3 -> Terminator2/1
  Controller Interface1/2 -> Terminator3/1
  Cable1/2 -> Subsystem3/1
  Cable2/1 -> Subsystem3/2

== system NCS_Simulation/Network/Ethernet (Ring) CAN/Consist 2 ==
  Burst Device : NCS_Library/Network/ETB/Burst Device  Address=[111 299]  Destination=[ 100 200]  Size=100  Port=1  ReplyAddress=[0 0]  Subscribe=[0 0; 0 0; 0 0; 0 0; 0 0]  msgType=Passive  T_x=0  Timeout=0  SDTv2=Disable  EnableToF=off  ToF=0  EnableBurst=off  ToB=0  Tx=0  number=1
  Burst Device1 : NCS_Library/Network/ETB/Burst Device  Address=[111 298]  Destination=[ 100 200]  Size=100  Port=1  ReplyAddress=[0 0]  Subscribe=[0 0; 0 0; 0 0; 0 0; 0 0]  msgType=Passive  T_x=0  Timeout=0  SDTv2=Disable  EnableToF=off  ToF=0  EnableBurst=off  ToB=0  Tx=0  number=1
  Cable{,1..3} (4 alike) : NCS_Library/Network/ETB/Cable  length=0  Cable=Coaxial
  ED : Subsystem  AncestorBlock=NCS_Library/Network/ETB/ED  mask{Address=[112 212], Destination=[112 211], Port=1, ReplyAddress=[0 0], Size=11, Subscribe=[112 211; 0 0; 0 0; 0 0; 0 0], msgType=Passive, Tx=0.1, Timeout=inf, SDTv2=Disable, EnableToF=off, ToF=6}
      mask prompts: Port "Destination Port"; ReplyAddress "Reply Address"; Size "Packet Size [Byte]"; Tx "Tx [ms]"; Timeout "TRDP Timeout [s]"; EnableToF "Enable Failure"; ToF "Time [s]"
      mask init:
      | if msgType == 3 || msgType == 4
      |     Tx = 0;
      | else
      |     Tx = Tx/1000;
      | end
      mask TypeOptions Port: 1 | 2 | 3 | 4 | 5 | 6 | 7 | 8 | Multicast
      mask TypeOptions msgType: Pull | Push cyclical | Push sporadic | Passive
      mask Callback msgType:
      | % Control parameter visiblity
      | % Disable Tx dialog, if it is not needed, because of a passive ED,
      | % which only receives.
      | 
      | % Get value
      | Modus = get_param(gcb,'msgType');
      | ToF = get_param(gcb,'EnableToF');
      | 
      | % Set the 'MaskVisibilities' property for each box
      | 
      | On = {'on','on','on','on','on','on','on','on','on','on','on','on'}; % Init
      | 
      | % Disable Tx Dialog, if not needed
      | 
      | if strcmp('Passive',Modus) || strcmp('Push Discrete',Modus)
      |     On{8} = 'off';
      | end
      | 
      | if strcmp('off',ToF)
      |     On{12} = 'off';
      | end
      | 
      | set_param(gcb,'MaskEnables',On );
      mask TypeOptions SDTv2: Disable | Enable
      mask Callback EnableToF:
      | % Control parameter visiblity
      | % Disable Tx dialog, if it is not needed, because of a passive ED,
      | % which only receives.
      | 
      | % Get value
      | Modus = get_param(gcb,'msgType');
      | ToF = get_param(gcb,'EnableToF');
      | 
      | % Set the 'MaskVisibilities' property for each box
      | 
      | On = {'on','on','on','on','on','on','on','on','on','on','on','on'}; % Init
      | 
      | % Disable Tx Dialog, if not needed
      | 
      | if strcmp('Passive',Modus) || strcmp('Push Discrete',Modus)
      |     On{8} = 'off';
      | end
      | 
      | if strcmp('off',ToF)
      |     On{12} = 'off';
      | end
      | 
      | set_param(gcb,'MaskEnables',On );
      mask DialogControl Container3 Prompt: Modus
      mask DialogControl Container4 Prompt: SDTv2
      mask DialogControl Container6 Prompt: Interrupts
      mask Display: disp([ 'End Device' '\n' get_param(gcb,'Address') ]);
  ED1 : NCS_Library/Network/ETB/ED  Address=[112 213]  Destination=[112 211]  Port=1  ReplyAddress=[0 0]  Size=11  Subscribe=[112 211; 0 0; 0 0; 0 0; 0 0]  msgType=Passive  Tx=0.1  Timeout=inf  SDTv2=Disable  EnableToF=off  ToF=0.5
  Ethernet_2-port_Switch : NCS_Library/Network/ETB/Ethernet_2-port_Switch  addstore=10  bandc=10^8  buffer_size=120000  cable_node=10  cable_LR=10
  Ethernet_2-port_Switch1 : NCS_Library/Network/ETB/Ethernet_2-port_Switch  addstore=10  bandc=10^8  buffer_size=120000  cable_node=10  cable_LR=10
  Ethernet_3-port_switch : NCS_Library/Network/ETB/Ethernet_3-port_switch  addstore=5  bandc=10^8  buffer_size=180000  cable_node=10  cable_L=10  cable_R=10
  Ethernet_3-port_switch1 : NCS_Library/Network/ETB/Ethernet_3-port_switch  addstore=5  bandc=10^8  buffer_size=180000  cable_node=10  cable_L=10  cable_R=10
  Ethernet_3-port_switch2 : NCS_Library/Network/ETB/Ethernet_3-port_switch  addstore=5  bandc=10^8  buffer_size=180000  cable_node=10  cable_L=10  cable_R=10
  Fieldbus 2 : Subsystem
  Output Control : Subsystem
  Redundant Device Control : Subsystem
  Terminator1 : Terminator
  Terminator3 : Terminator
  out2 : Outport
  wires:
  Fieldbus 2/2(U) -> Output Control/3(U)  "U"
  ED/2(ReceivedData) -> Output Control/2(Y_M1)  "Y_M"
  Cable3/2 -> Ethernet_2-port_Switch1/1
  Cable2/1 -> Ethernet_3-port_switch1/1
  ED1/1 -> Redundant Device Control/2(InTx)
  Ethernet_2-port_Switch/2 -> Burst Device/1
  Cable2/2 -> Ethernet_3-port_switch2/2
  Ethernet_2-port_Switch1/1 -> Cable3/1
  Burst Device/1 -> Ethernet_2-port_Switch/2
  Ethernet_3-port_switch/3 -> ED/1(RxFromBus)
  Cable/1 -> Ethernet_2-port_Switch/1
  ED/4(Failed) -> Redundant Device Control/1(<#Receive>), Output Control/1(<#Receive>)
  Cable1/1 -> Ethernet_3-port_switch/1
  Burst Device1/1 -> Ethernet_2-port_Switch1/2
  Ethernet_3-port_switch2/3 -> ED1/1
  Fieldbus 2/1(OutToEthernet) -> Ethernet_3-port_switch1/3
  Ethernet_3-port_switch1/3 -> Fieldbus 2/1(InFromEthernet)
  Ethernet_2-port_Switch1/2 -> Burst Device1/1
  Ethernet_3-port_switch2/1 -> Cable2/1
  ED1/3 -> Output Control/4(Y_M2)  "Y_M"
  Redundant Device Control/1(OutTx) -> Ethernet_3-port_switch2/3
  Ethernet_3-port_switch/1 -> Cable/1
  Cable3/1 -> Ethernet_3-port_switch2/1
  Output Control/1(Out1) -> out2/1
  Ethernet_3-port_switch2/2 -> Cable3/2
  Ethernet_3-port_switch1/2 -> Cable2/2
  Ethernet_3-port_switch/2 -> Cable1/2
  Cable/2 -> Ethernet_3-port_switch/2
  Ethernet_2-port_Switch/1 -> Cable/2
  Cable1/2 -> Ethernet_3-port_switch1/2
  Ethernet_3-port_switch1/1 -> Cable1/1
  ED1/2 -> Terminator1/1
  ED/1(TxToBus) -> Ethernet_3-port_switch/3
  [U_2] -> ED/2(Signal)  "U"
  [U_2] -> ED1/2  "U"
  ED/3(Recorder) -> Terminator3/1

== system NCS_Simulation/Network/Ethernet (Line)/Consist 1/Output Control ==
  Failed : Inport
  Y_M1 : Inport  Port=2
  U : Inport  Port=3
  Y_M2 : Inport  Port=4
  Logical Operator : Logic  Operator=NOT  AllPortsSameDT=off  OutDataTypeStr=boolean
  Mux : NCS_Library/Network/Applications/Multiplexer/Mux  SystemSampleTime=-1
  Switch : Switch  Criteria=u2 > Threshold
  Out1 : Outport
  wires:
  Y_M2/1 -> Switch/3
  Logical Operator/1 -> Switch/2
  Y_M1/1 -> Switch/1
  Switch/1 -> Mux/1
  U/1 -> Mux/2
  Failed/1 -> Logical Operator/1
  Mux/1 -> Out1/1

== system NCS_Simulation/Network/Ethernet (Line)/Consist 1/Redundant Device Control ==
  Failed : Inport
  InTx : Inport  Port=2
  Add Constant : Bias  Bias=1
  Display : Display
  Entity Output Switch : EntityOutputSwitch  InputPortMessageModes=m,m  OutputPortMessageModes=m,m  SwitchingCriterion=From control port  SwitchAttributeName=Attribute1
      settings: InputPortMap=u0,u1
  Message Send : MessageSend  OutputPortMessageModes=m
      settings: InputPortMap=u1
  No Failure : EntityTerminator  InputPortMessageModes=m  NumberEntitiesArrived=on
      settings: OutputPortMap=o0
  OutTx : Outport
  wires:
  Entity Output Switch/2 -> OutTx/1
  InTx/1 -> Entity Output Switch/2
  Entity Output Switch/1 -> No Failure/1
  No Failure/1 -> Display/1
  Failed/1 -> Add Constant/1
  Add Constant/1 -> Message Send/1
  Message Send/1 -> Entity Output Switch/1

== system NCS_Simulation/Network/Ethernet (Line)/Consist 2/Output Control ==
  Failed : Inport
  Y_M1 : Inport  Port=2
  U : Inport  Port=3
  Y_M2 : Inport  Port=4
  Logical Operator : Logic  Operator=NOT  AllPortsSameDT=off  OutDataTypeStr=boolean
  Mux : NCS_Library/Network/Applications/Multiplexer/Mux  SystemSampleTime=-1
  Switch : Switch  Criteria=u2 > Threshold
  Out1 : Outport
  wires:
  Y_M2/1 -> Switch/3
  Logical Operator/1 -> Switch/2
  Y_M1/1 -> Switch/1
  Switch/1 -> Mux/1
  U/1 -> Mux/2
  Failed/1 -> Logical Operator/1
  Mux/1 -> Out1/1

== system NCS_Simulation/Network/Ethernet (Line)/Consist 2/Redundant Device Control ==
  Failed : Inport
  InTx : Inport  Port=2
  Add Constant : Bias  Bias=1
  Display : Display
  Entity Output Switch : EntityOutputSwitch  InputPortMessageModes=m,m  OutputPortMessageModes=m,m  SwitchingCriterion=From control port  SwitchAttributeName=Attribute1
      settings: InputPortMap=u0,u1
  Message Send : MessageSend  OutputPortMessageModes=m
      settings: InputPortMap=u1
  No Failure : EntityTerminator  InputPortMessageModes=m  NumberEntitiesArrived=on
      settings: OutputPortMap=o0
  OutTx : Outport
  wires:
  Entity Output Switch/2 -> OutTx/1
  InTx/1 -> Entity Output Switch/2
  Entity Output Switch/1 -> No Failure/1
  No Failure/1 -> Display/1
  Failed/1 -> Add Constant/1
  Add Constant/1 -> Message Send/1
  Message Send/1 -> Entity Output Switch/1
